simulink model "HSX_double_fin2"  (R2023b)
settings: Solver=VariableStepAuto  StartTime=0.0  StopTime=T_end  RelTol=1e-3
values from neighbouring files (symbols this model uses):
  Kaa = 0    [fin.m]
  Kanti = 0.95    [fin.m]
  Ki = K*Rtot    (= 45.48)    [fin.m]
  Kii = 0.001    [fin.m]
  Kp = K*Ltot    (= 10.10125)    [fin.m]
  Kpp = 0.01    [fin.m]
  Lc = 100e-6    (= 0.0001)    [fin.m]
  LHSX = 0.02    [fin.m]
  Ltot = 10*LHSX+La+Lc/n    (= 0.202025)    [fin.m]
  multi_enable = 1    [fin.m]
  n = 4    [fin.m]
  Ra = 0.0096    [fin.m]
  RHSX = 0.09    [fin.m]
  T_trigger = 15    [fin.m]
  Tdead = Ts/100    (= 1e-06)    [fin.m]
  Ts = 1/fs    (= 0.0001)    [fin.m]
  Tsamp = 1/fsamp    (= 2e-05)    [fin.m]
  VDC = 40    [fin.m]
  Vf = 3.1    [fin.m]
libraries: spsCurrentMeasurementLib x6, spsVoltageMeasurementLib x6, spsSeriesRLCBranchLib x6, spsTriangleGeneratorLib x4, spsMosfetLib x4, spsControlledVoltageSourceLib x2, spsDCMachineLib x2, spsGroundLib x2, spsIdealSwitchLib x2, spsDCVoltageSourceLib x2, spsDiodeLib x1, sps_lib x1
settings Model: Creator=baik3-ad  LastModifiedBy=Hyeongmeen

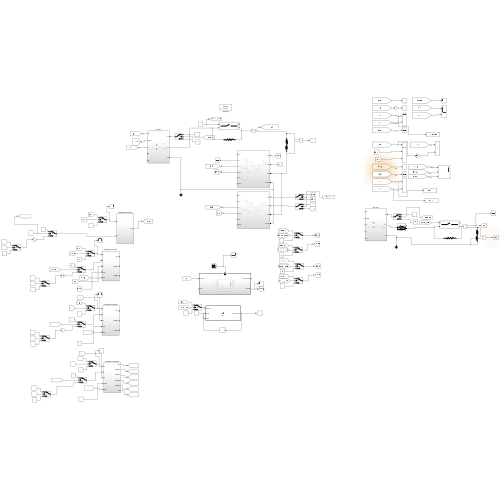
[thumbnail: Simulink's stored preview of the top-level diagram]
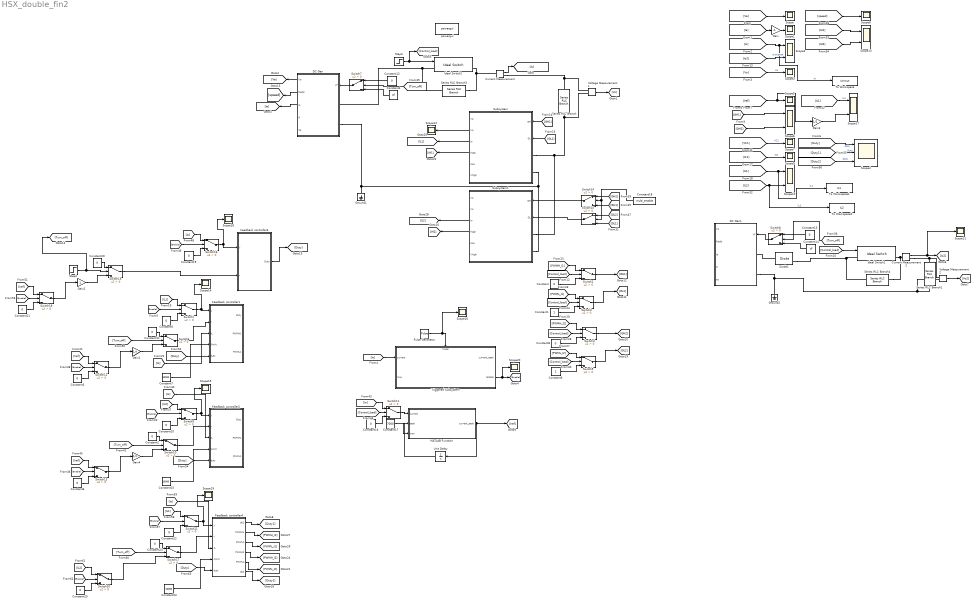
== system HSX_double_fin2 ==
  Constant{,2..3,5..6,8,10..13,16,19..22,24..25} (17 alike) : Constant  Value=0
  Constant1 : Constant
  Constant14 : Constant  Value=Vf
  Constant15 : Constant  Value=10000
  Constant17 : Constant  Value=7000
  Constant18 : Constant  Value=multi_enable
  Constant23 : Constant  Value=10000
  Constant4 : Constant  Value=Vf
  Constant7 : Constant  Value=10000
  Constant9 : Constant
  Current Measurement : spsCurrentMeasurementLib/Current Measurement  PhasorSimulation=off  OutputType=Complex  PSBequivalent=0
  Current Measurement2 : spsCurrentMeasurementLib/Current Measurement  PhasorSimulation=off  OutputType=Complex  PSBequivalent=0
  DC Gen : Subsystem
  DC Gen1 : Subsystem
  Diode1 : spsDiodeLib/Diode  Ron=0.001  Lon=0  Vf=0.8  IC=0  UseSnubber=0  Rs=500  Cs=250e-9  Measurements=on
  Feedback controller1 : Subsystem
  Feedback controller2 : Subsystem
  Feedback controller3 : Subsystem
  Feedback controller4 : Subsystem
  Gain : Gain  Gain=-1
  Gain1 : Gain  Gain=1/n
  Gain2 : Gain
  Gain3 : Gain  Gain=1/2
  Gain4 : Gain  Gain=1/n
  Ground1 : spsGroundLib/Ground  LConnTagsString=a
  Ground2 : spsGroundLib/Ground  LConnTagsString=a
  Ideal Switch1 : spsIdealSwitchLib/Ideal Switch  Ron=1e-6  Lon=0  IC=0  Rs=1e8  Cs=0  Measurements=on
  Ideal Switch2 : spsIdealSwitchLib/Ideal Switch  Ron=1e-6  Lon=0  IC=0  Rs=1e8  Cs=0  Measurements=on
  MATLAB Function : MATLAB Function  TreatAsAtomicUnit=on
  Pulse Generator : DiscretePulseGenerator  PulseType=Time based  Period=Ts  PulseWidth=50
  Scope{,1,3,5,7..9,11..12,14..16,18..20} (15 alike) : Scope
  Scope{2,6,10,13,17} (5 alike) : Scope  NumInputPorts=2
  Scope4 : Scope  NumInputPorts=3
  Series RLC Branch : spsSeriesRLCBranchLib/Series RLC Branch  LConnTagsString=__new0  RConnTagsString=__new0  BranchType=RL  Resistance=RHSX*10  Inductance=LHSX*10  SetiL0=off  InitialCurrent=0  Capacitance=1e-6  Setx0=off  InitialVoltage=0  Measurements=None
  Series RLC Branch1 : spsSeriesRLCBranchLib/Series RLC Branch  LConnTagsString=__new0  RConnTagsString=__new0  BranchType=RL  Resistance=RHSX*10  Inductance=LHSX*10  SetiL0=off  InitialCurrent=0  Capacitance=1e-6  Setx0=off  InitialVoltage=0  Measurements=None
  Series RLC Branch3 : spsSeriesRLCBranchLib/Series RLC Branch  LConnTagsString=__new0  RConnTagsString=__new0  BranchType=R  Resistance=1e8  Inductance=0  SetiL0=off  InitialCurrent=0  Capacitance=1e-6  Setx0=off  InitialVoltage=0  Measurements=None
  Series RLC Branch4 : spsSeriesRLCBranchLib/Series RLC Branch  LConnTagsString=__new0  RConnTagsString=__new0  BranchType=R  Resistance=1e8  Inductance=0  SetiL0=off  InitialCurrent=0  Capacitance=1e-6  Setx0=off  InitialVoltage=0  Measurements=None
  Step2 : Step  Time=T_trigger+1.5  SampleTime=0  VectorParams1D=off  ZeroCross=off
  Step3 : Step  Time=T_trigger  SampleTime=0  VectorParams1D=off  ZeroCross=off
  Subsystem : Subsystem
  Subsystem1 : Subsystem
  Switch{1..21} (21 alike) : Switch  Criteria=u2 > Threshold  SaturateOnIntegerOverflow=off  InputSameDT=off
  To Workspace : ToWorkspace  VariableName=simout  SaveFormat=Timeseries  SampleTime=-1
  To Workspace1 : ToWorkspace  VariableName=IL1  SaveFormat=Timeseries  SampleTime=-1
  To Workspace2 : ToWorkspace  VariableName=IL2  SaveFormat=Timeseries  SampleTime=-1
  Triggered Subsystem : Subsystem  TreatAsAtomicUnit=on
  Unit Delay : UnitDelay  SampleTime=-1  HasFrameUpgradeWarning=on
  Voltage Measurement1 : spsVoltageMeasurementLib/Voltage Measurement  PhasorSimulation=off  OutputType=Complex  PSBequivalent=0
  Voltage Measurement2 : spsVoltageMeasurementLib/Voltage Measurement  PhasorSimulation=off  OutputType=Complex  PSBequivalent=0
  powergui : sps_lib/powergui  Priority=1  SimulationMode=Discrete  SampleTime=Tsamp  frequency=60  Iterations=50  frequencyindice=0  Pbase=100e6  ErrMax=1e-4  UnitsV=kV  UnitsW=MW  buscounter=0  FunctionMessages=off  echomessages=off  EnableUseOfTLC=off  CurrentSourceSwitches=off  DisableSnubberDevices=off  DisableRonSwitches=off  DisableVfSwitches=off  DisplayEquations=off  AutomaticDiscreteSolvers=off  SolverType=Tustin/Backward Euler (TBE)  Interpol=off  ExternalGateDelay=off  methode=off  Ts=100  x0status=blocks  SPID=on  SwTol=0  HookPort=off  NonlinearTolerance=1e-4  nMaxIteration=100  ContinueOnMaxIteration=off  RestoreLinks=warning  ResistiveCurrentMeasurement=off  Frange=[0:2:500]  Ylog=off  Xlog=on  ShowGrid=off  save=off  variable=ZData  structure=0  ZoomFFT=off  StartTime=0.0  cycles=1  DisplayStyle=1  fundamental=60  FreqAxis=off  MaxFrequency=1000  frequencyindicesteady=1  RmsSteady=1  display=off
  wires:
  Step3/1 -> [Control_load], Ideal Switch2/1
  Current Measurement/1 -> [Io]
  Voltage Measurement1/1 -> [Vo]
  [Va] -> Scope/1
  [Io] -> To Workspace/1, Scope2/1  "Io"
  [Vo] -> Scope3/1  "Vo"
  [Ia] -> Gain/1
  Gain/1 -> Scope1/1
  [Iref] -> Gain3/1, Scope5/1
  [VC1] -> Scope7/1  "VC1"
  Switch2/1 -> [GH1]
  Switch3/1 -> [GL1]
  [speed] -> Scope8/1
  [IC1] -> Scope9/1  "IC1"
  [IL1] -> To Workspace1/1, Scope10/1  "IL1"
  [Enable] -> Switch1/2
  Constant5/1 -> Switch1/3
  [IL1] -> Switch1/1
  Switch1/1 -> Feedback controller1/1(y), Scope14/1
  Switch6/1 -> Feedback controller1/2(r)
  [Control_load] -> Switch2/2
  [PWMH_I1] -> Switch2/1
  Constant/1 -> Switch2/3
  [PWML_I1] -> Switch3/1
  Constant1/1 -> Switch3/3
  [Control_load] -> Switch3/2
  Current Measurement2/1 -> Scope11/1, [Io2]
  Voltage Measurement2/1 -> [Vo2]
  [Control_load] -> Ideal Switch1/1
  [Io2] -> Scope2/2  "Io original"
  [Io] -> Feedback controller1/3(IL)
  Constant7/1 -> Feedback controller1/4(Ilimit)
  Switch7/1 -> DC Gen/1(Vf)
  Subsystem/3(Io) -> [IL1]
  Subsystem/2(Vo) -> Scope12/1
  DC Gen/3(Ia) -> [Ia]
  DC Gen/1(Va) -> [Va]
  DC Gen/2(Rad/s) -> [speed]
  Switch4/1 -> [GH2]
  [Control_load] -> Switch5/2
  Constant9/1 -> Switch5/3
  [Control_load] -> Switch4/2
  [PWML_I2] -> Switch5/1
  [PWMH_I2] -> Switch4/1
  Constant8/1 -> Switch4/3
  Switch5/1 -> [GL2]
  [GH1] -> Subsystem/1(GH)
  [IL2] -> To Workspace2/1, Scope10/2  "IL2"
  [IH1] -> Scope13/1
  [IH2] -> Scope13/2
  Subsystem/4(Ihigh) -> [IH1]
  [Turn_off] -> Switch6/2
  Constant11/1 -> Switch6/1
  Constant4/1 -> Switch7/3
  [Turn_off] -> Switch7/2
  Constant12/1 -> Switch7/1
  Constant13/1 -> Switch8/1
  Constant14/1 -> Switch8/3
  [Turn_off] -> Switch8/2
  Switch8/1 -> DC Gen1/1(Vf)
  Switch14/1 -> Subsystem1/1(GH)
  Subsystem1/3(Io) -> [IL2]
  Subsystem1/4(Ihigh) -> [IH2]
  Constant2/1 -> Switch10/1
  [Io] -> Feedback controller2/3(IL)
  Switch9/1 -> Scope15/1, Feedback controller2/1(y)
  [Turn_off] -> Switch10/2
  Constant15/1 -> Feedback controller2/4(Ilimit)
  Switch10/1 -> Feedback controller2/2(r)
  [Enable] -> Switch9/2
  Constant10/1 -> Switch9/3
  [IL2] -> Switch9/1
  Switch12/1 -> Gain1/1
  Gain1/1 -> Switch6/3
  Gain4/1 -> Switch10/3
  Pulse Generator/1 -> Scope16/1, Triggered Subsystem/Trigger
  [IL1] -> Scope17/1  "IL1"
  Gain3/1 -> Scope17/2
  [Control_load] -> Switch11/2
  [Io] -> Switch11/1
  Constant17/1 -> MATLAB Function/3(max)
  Constant16/1 -> Switch11/3
  Switch11/1 -> MATLAB Function/1(current)
  MATLAB Function/1(current_peak) -> Unit Delay/1, [Iref]
  Unit Delay/1 -> MATLAB Function/2(peak)
  [Io] -> Triggered Subsystem/1(current)
  Triggered Subsystem/2(Enable) -> Scope20/1, [Enable]
  [Enable] -> Switch12/2
  [Iref] -> Switch12/1
  Constant3/1 -> Switch12/3
  Constant6/1 -> Switch13/3
  [Iref] -> Switch13/1
  [Enable] -> Switch13/2
  Switch13/1 -> Gain4/1
  Switch15/1 -> Subsystem1/2(GL)
  [GL1] -> Subsystem/2(GL)
  [GH1] -> Scope6/1
  [GH2] -> Scope6/2
  [GH2] -> Switch14/1
  [GL2] -> Switch15/1
  [GH1] -> Switch14/3
  [GL1] -> Switch15/3
  Constant18/1 -> Switch15/2, Switch14/2
  [Enable] -> Switch16/2
  [Io] -> Switch16/1
  Switch16/1 -> Feedback controller3/1(y), Scope18/1
  Constant19/1 -> Switch16/3
  Switch19/1 -> Feedback controller3/2(r)
  [Enable] -> Switch18/2
  Constant21/1 -> Switch18/3
  Gain2/1 -> Switch19/3
  Switch18/1 -> Gain2/1
  [Iref] -> Switch18/1
  Step2/1 -> [Turn_off], Switch19/2
  Constant20/1 -> Switch19/1
  Feedback controller3/1(Duty) -> [Duty]
  [Duty] -> Feedback controller1/5(duty)
  [Duty] -> Feedback controller2/5(duty)
  [Duty] -> Scope4/1  "Duty"
  [Duty1] -> Scope4/2  "Duty"
  [Duty2] -> Scope4/3  "Duty"
  Constant24/1 -> Switch17/1
  [Turn_off] -> Switch17/2
  Constant25/1 -> Switch20/3
  Switch20/1 -> Switch17/3
  [Duty] -> Feedback controller4/5(duty)
  [Enable] -> Switch20/2
  [IL2] -> Switch20/1
  Constant23/1 -> Feedback controller4/4(Ilimit)
  Constant22/1 -> Switch21/3
  [IL1] -> Switch21/1
  Switch21/1 -> Scope19/1, Feedback controller4/1(y)
  Switch17/1 -> Feedback controller4/2(r)
  [Enable] -> Switch21/2
  [Io] -> Feedback controller4/3(IL)
  Feedback controller4/4(PWMH2) -> [PWMH_I2]
  Feedback controller4/5(PWML2) -> [PWML_I2]
  Feedback controller4/3(PWML1) -> [PWML_I1]
  Feedback controller4/2(PWMH1) -> [PWMH_I1]
  Feedback controller4/1(do1) -> [Duty1]
  Feedback controller4/6(do2) -> [Duty2]
  connections:
  DC Gen/LConn2 -- Subsystem1/LConn2 -- Subsystem/LConn2 -- Ground1/LConn1
  Current Measurement/RConn1 -- Voltage Measurement1/LConn1 -- Series RLC Branch/LConn1
  Current Measurement/LConn1 -- Ideal Switch2/RConn1 -- Series RLC Branch3/LConn1
  Ideal Switch1/LConn1 -- Diode1/RConn1 -- Series RLC Branch4/RConn1
  Ideal Switch1/RConn1 -- Current Measurement2/LConn1 -- Series RLC Branch4/LConn1
  Series RLC Branch1/LConn1 -- Voltage Measurement2/LConn1 -- Current Measurement2/RConn1
  Diode1/LConn1 -- DC Gen1/LConn1
  DC Gen1/LConn2 -- Series RLC Branch1/RConn1 -- Voltage Measurement2/LConn2 -- Ground2/LConn1
  Ideal Switch2/LConn1 -- DC Gen/LConn1 -- Series RLC Branch3/RConn1
  Voltage Measurement1/LConn2 -- Subsystem1/LConn1 -- Subsystem/LConn1 -- Series RLC Branch/RConn1

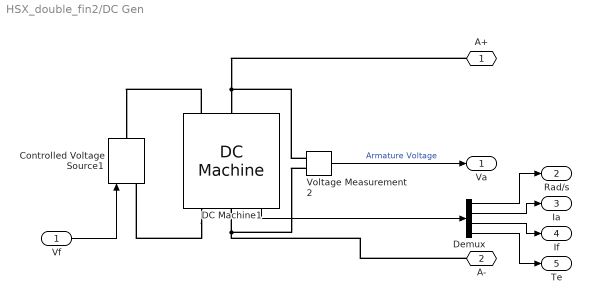
== system HSX_double_fin2/DC Gen ==
  Vf : Inport
  Controlled Voltage Source1 : spsControlledVoltageSourceLib/Controlled Voltage Source  Initialize=on  Source_Type=DC  Amplitude=0  Phase=0  Frequency=0  Measurements=Voltage
  DC Machine1 : spsDCMachineLib/DC Machine  PresetModel=No  MechanicalLoad=Torque TL  FieldType=Wound  ShowDetailedParameters=on  MeasurementBus=off  RLa="[Ra  0.002]"  RLf=[0.0054 0.0125]  Laf=Laf  MachineConstant=Torque constant (N.m/A)  Ke=1.8  Kt=1.8  J=137  Bm=0  Tf=0  w0=w_initial  Ifinit=0  TsPowergui=0  TsBlock=-1
  Demux : Demux
  Voltage Measurement2 : spsVoltageMeasurementLib/Voltage Measurement  PhasorSimulation=off  OutputType=Complex  PSBequivalent=0
  A+ : PMIOPort  Side=Left
  A- : PMIOPort  Port=2  Side=Left
  Va : Outport
  Rad/s : Outport  Port=2
  Ia : Outport  Port=3
  If : Outport  Port=4
  Te : Outport  Port=5
  wires:
  DC Machine1/1 -> Demux/1
  Vf/1 -> Controlled Voltage Source1/1
  Voltage Measurement2/1 -> Va/1  "Armature Voltage"
  Demux/1 -> Rad/s/1
  Demux/4 -> Te/1
  Demux/3 -> If/1
  Demux/2 -> Ia/1
  connections:
  Voltage Measurement2/LConn1 -- A+/RConn1 -- DC Machine1/LConn1
  A-/RConn1 -- Voltage Measurement2/LConn2 -- DC Machine1/RConn1
  DC Machine1/LConn2 -- Controlled Voltage Source1/RConn1
  DC Machine1/RConn2 -- Controlled Voltage Source1/LConn1

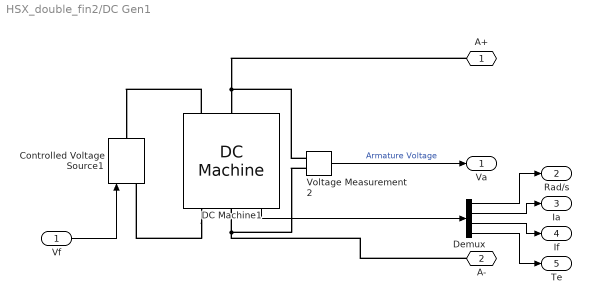
== system HSX_double_fin2/DC Gen1 ==
  Vf : Inport
  Controlled Voltage Source1 : spsControlledVoltageSourceLib/Controlled Voltage Source  Initialize=on  Source_Type=DC  Amplitude=0  Phase=0  Frequency=0  Measurements=Voltage
  DC Machine1 : spsDCMachineLib/DC Machine  PresetModel=No  MechanicalLoad=Torque TL  FieldType=Wound  ShowDetailedParameters=on  MeasurementBus=off  RLa="[Ra  0.002]"  RLf=[0.0054 0.0125]  Laf=Laf  MachineConstant=Torque constant (N.m/A)  Ke=1.8  Kt=1.8  J=137  Bm=0  Tf=0  w0=w_initial  Ifinit=0  TsPowergui=0  TsBlock=-1
  Demux : Demux
  Voltage Measurement2 : spsVoltageMeasurementLib/Voltage Measurement  PhasorSimulation=off  OutputType=Complex  PSBequivalent=0
  A+ : PMIOPort  Side=Left
  A- : PMIOPort  Port=2  Side=Left
  Va : Outport
  Rad/s : Outport  Port=2
  Ia : Outport  Port=3
  If : Outport  Port=4
  Te : Outport  Port=5
  wires:
  DC Machine1/1 -> Demux/1
  Vf/1 -> Controlled Voltage Source1/1
  Voltage Measurement2/1 -> Va/1  "Armature Voltage"
  Demux/1 -> Rad/s/1
  Demux/4 -> Te/1
  Demux/3 -> If/1
  Demux/2 -> Ia/1
  connections:
  Voltage Measurement2/LConn1 -- A+/RConn1 -- DC Machine1/LConn1
  A-/RConn1 -- Voltage Measurement2/LConn2 -- DC Machine1/RConn1
  DC Machine1/LConn2 -- Controlled Voltage Source1/RConn1
  DC Machine1/RConn2 -- Controlled Voltage Source1/LConn1

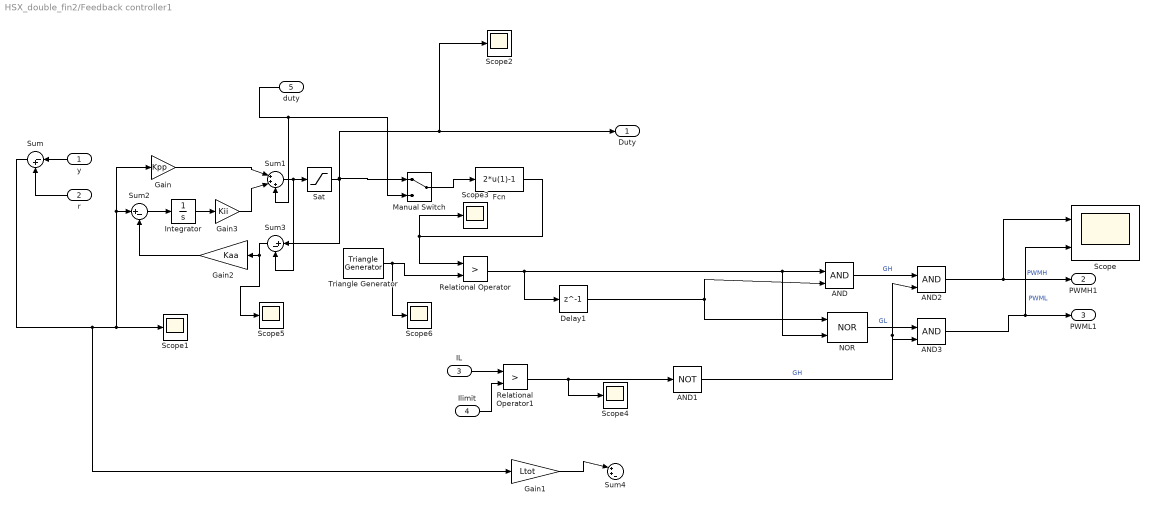
== system HSX_double_fin2/Feedback controller1 ==
  y : Inport
  r : Inport  Port=2
  IL : Inport  Port=3
  Ilimit : Inport  Port=4
  duty : Inport  Port=5
  AND : Logic  IconShape=distinctive  AllPortsSameDT=off  OutDataTypeStr=boolean
  AND1 : Logic  Operator=NOT  IconShape=distinctive  AllPortsSameDT=off  OutDataTypeStr=boolean
  AND2 : Logic  IconShape=distinctive  AllPortsSameDT=off  OutDataTypeStr=boolean
  AND3 : Logic  IconShape=distinctive  AllPortsSameDT=off  OutDataTypeStr=boolean
  Delay1 : Delay  DelayLength=1  InitialCondition=0  SampleTime=Tdead
  Fcn : Fcn  Expr=2*u(1)-1
  Gain : Gain  Gain=Kpp
  Gain1 : Gain  Gain=Ltot
  Gain2 : Gain  Gain=Kaa
  Gain3 : Gain  Gain=Kii
  Integrator : Integrator
  Manual Switch : ManualSwitch
  NOR : Logic  Operator=NOR  IconShape=distinctive  AllPortsSameDT=off
  Relational Operator : RelationalOperator  Operator=>  OutDataTypeStr=boolean  RndMeth=Simplest  InputSameDT=off
  Relational Operator1 : RelationalOperator  Operator=>  OutDataTypeStr=boolean  RndMeth=Simplest  InputSameDT=off
  Sat : Saturate  UpperLimit=1  LowerLimit=0
  Scope : Scope  NumInputPorts=2
  Scope{1..6} (6 alike) : Scope
  Sum : Sum  Inputs=|-+  InputSameDT=on  SaturateOnIntegerOverflow=on  OutDataTypeStr=Inherit: Same as first input
  Sum1 : Sum  Inputs=|+++
  Sum2 : Sum  Inputs=|+-
  Sum3 : Sum  Inputs=|+-
  Sum4 : Sum  Inputs=|++-
  Triangle Generator : spsTriangleGeneratorLib/Triangle Generator  Freq=1/Ts  Phase=0  Ts=Tsamp
  Duty : Outport  VectorParamsAs1DForOutWhenUnconnected=off
  PWMH1 : Outport  Port=2  VectorParamsAs1DForOutWhenUnconnected=off
  PWML1 : Outport  Port=3  VectorParamsAs1DForOutWhenUnconnected=off
  wires:
  Sum/1 -> Gain1/1, Scope1/1, Gain/1, Sum2/1
  y/1 -> Sum/1
  r/1 -> Sum/2
  Sat/1 -> Sum3/1, Manual Switch/1, Scope2/1, Duty/1
  Sum1/1 -> Sum3/2, Sat/1
  Gain/1 -> Sum1/1
  Sum2/1 -> Integrator/1
  Sum3/1 -> Scope5/1, Gain2/1
  Gain2/1 -> Sum2/2
  Triangle Generator/1 -> Scope6/1, Relational Operator/2
  Relational Operator/1 -> Delay1/1, NOR/2, AND/1
  Delay1/1 -> NOR/1, AND/2
  Fcn/1 -> Scope3/1, Relational Operator/1
  Integrator/1 -> Gain3/1
  Gain3/1 -> Sum1/2
  IL/1 -> Relational Operator1/1
  Ilimit/1 -> Relational Operator1/2
  AND/1 -> AND2/1  "GH"
  AND2/1 -> Scope/1, PWMH1/1  "PWMH"
  AND3/1 -> PWML1/1, Scope/2  "PWML"
  NOR/1 -> AND3/1  "GL"
  Relational Operator1/1 -> Scope4/1, AND1/1
  AND1/1 -> AND3/2, AND2/2  "GH"
  Manual Switch/1 -> Fcn/1
  Gain1/1 -> Sum4/1
  duty/1 -> Sum1/3, Manual Switch/2

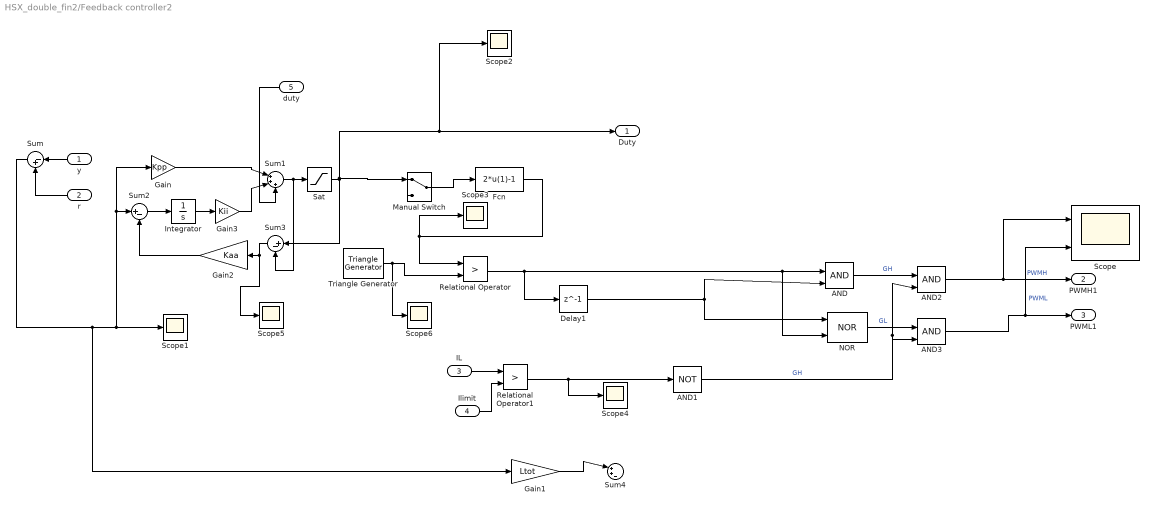
== system HSX_double_fin2/Feedback controller2 ==
  y : Inport
  r : Inport  Port=2
  IL : Inport  Port=3
  Ilimit : Inport  Port=4
  duty : Inport  Port=5
  AND : Logic  IconShape=distinctive  AllPortsSameDT=off  OutDataTypeStr=boolean
  AND1 : Logic  Operator=NOT  IconShape=distinctive  AllPortsSameDT=off  OutDataTypeStr=boolean
  AND2 : Logic  IconShape=distinctive  AllPortsSameDT=off  OutDataTypeStr=boolean
  AND3 : Logic  IconShape=distinctive  AllPortsSameDT=off  OutDataTypeStr=boolean
  Delay1 : Delay  DelayLength=1  InitialCondition=0  SampleTime=Tdead
  Fcn : Fcn  Expr=2*u(1)-1
  Gain : Gain  Gain=Kpp
  Gain1 : Gain  Gain=Ltot
  Gain2 : Gain  Gain=Kaa
  Gain3 : Gain  Gain=Kii
  Integrator : Integrator
  Manual Switch : ManualSwitch
  NOR : Logic  Operator=NOR  IconShape=distinctive  AllPortsSameDT=off
  Relational Operator : RelationalOperator  Operator=>  OutDataTypeStr=boolean  RndMeth=Simplest  InputSameDT=off
  Relational Operator1 : RelationalOperator  Operator=>  OutDataTypeStr=boolean  RndMeth=Simplest  InputSameDT=off
  Sat : Saturate  UpperLimit=1  LowerLimit=0
  Scope : Scope  NumInputPorts=2
  Scope{1..6} (6 alike) : Scope
  Sum : Sum  Inputs=|-+  InputSameDT=on  SaturateOnIntegerOverflow=on  OutDataTypeStr=Inherit: Same as first input
  Sum1 : Sum  Inputs=|+++
  Sum2 : Sum  Inputs=|+-
  Sum3 : Sum  Inputs=|+-
  Sum4 : Sum  Inputs=|++-
  Triangle Generator : spsTriangleGeneratorLib/Triangle Generator  Freq=1/Ts  Phase=180  Ts=Tsamp
  Duty : Outport  VectorParamsAs1DForOutWhenUnconnected=off
  PWMH1 : Outport  Port=2  VectorParamsAs1DForOutWhenUnconnected=off
  PWML1 : Outport  Port=3  VectorParamsAs1DForOutWhenUnconnected=off
  wires:
  Sum/1 -> Gain1/1, Scope1/1, Gain/1, Sum2/1
  y/1 -> Sum/1
  r/1 -> Sum/2
  Sat/1 -> Sum3/1, Manual Switch/1, Scope2/1, Duty/1
  Sum1/1 -> Sum3/2, Sat/1
  Gain/1 -> Sum1/1
  Sum2/1 -> Integrator/1
  Sum3/1 -> Scope5/1, Gain2/1
  Gain2/1 -> Sum2/2
  Triangle Generator/1 -> Scope6/1, Relational Operator/2
  Relational Operator/1 -> Delay1/1, NOR/2, AND/1
  Delay1/1 -> NOR/1, AND/2
  Fcn/1 -> Scope3/1, Relational Operator/1
  Integrator/1 -> Gain3/1
  Gain3/1 -> Sum1/2
  IL/1 -> Relational Operator1/1
  Ilimit/1 -> Relational Operator1/2
  AND/1 -> AND2/1  "GH"
  AND2/1 -> Scope/1, PWMH1/1  "PWMH"
  AND3/1 -> PWML1/1, Scope/2  "PWML"
  NOR/1 -> AND3/1  "GL"
  Relational Operator1/1 -> Scope4/1, AND1/1
  AND1/1 -> AND3/2, AND2/2  "GH"
  Manual Switch/1 -> Fcn/1
  Gain1/1 -> Sum4/1
  duty/1 -> Sum1/3

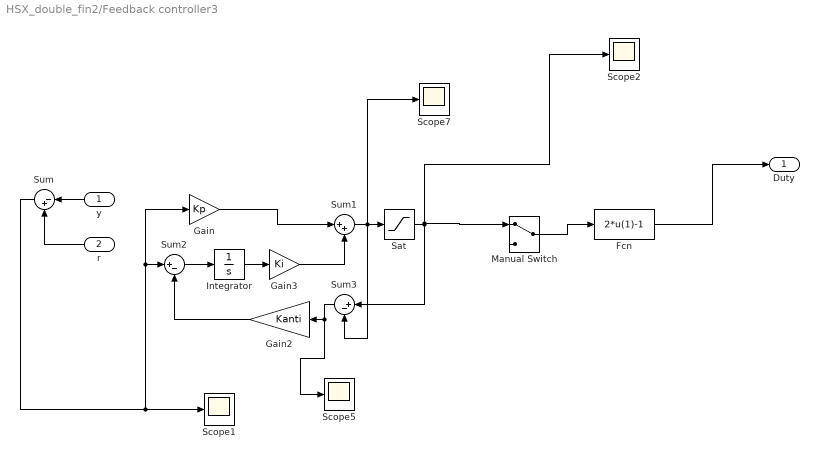
== system HSX_double_fin2/Feedback controller3 ==
  y : Inport
  r : Inport  Port=2
  Fcn : Fcn  Expr=2*u(1)-1
  Gain : Gain  Gain=Kp
  Gain2 : Gain  Gain=Kanti
  Gain3 : Gain  Gain=Ki
  Integrator : Integrator
  Manual Switch : ManualSwitch
  Sat : Saturate  UpperLimit=1  LowerLimit=0
  Scope{1..2,5,7} (4 alike) : Scope
  Sum : Sum  Inputs=|-+  InputSameDT=on  SaturateOnIntegerOverflow=on  OutDataTypeStr=Inherit: Same as first input
  Sum1 : Sum  Inputs=|++
  Sum2 : Sum  Inputs=|+-
  Sum3 : Sum  Inputs=|+-
  Duty : Outport  VectorParamsAs1DForOutWhenUnconnected=off
  wires:
  Sum/1 -> Scope1/1, Gain/1, Sum2/1
  y/1 -> Sum/1
  r/1 -> Sum/2
  Sat/1 -> Sum3/1, Manual Switch/1, Scope2/1
  Gain/1 -> Sum1/1
  Sum2/1 -> Integrator/1
  Sum3/1 -> Scope5/1, Gain2/1
  Gain2/1 -> Sum2/2
  Integrator/1 -> Gain3/1
  Gain3/1 -> Sum1/2
  Manual Switch/1 -> Fcn/1
  Sum1/1 -> Scope7/1, Sat/1, Sum3/2
  Fcn/1 -> Duty/1

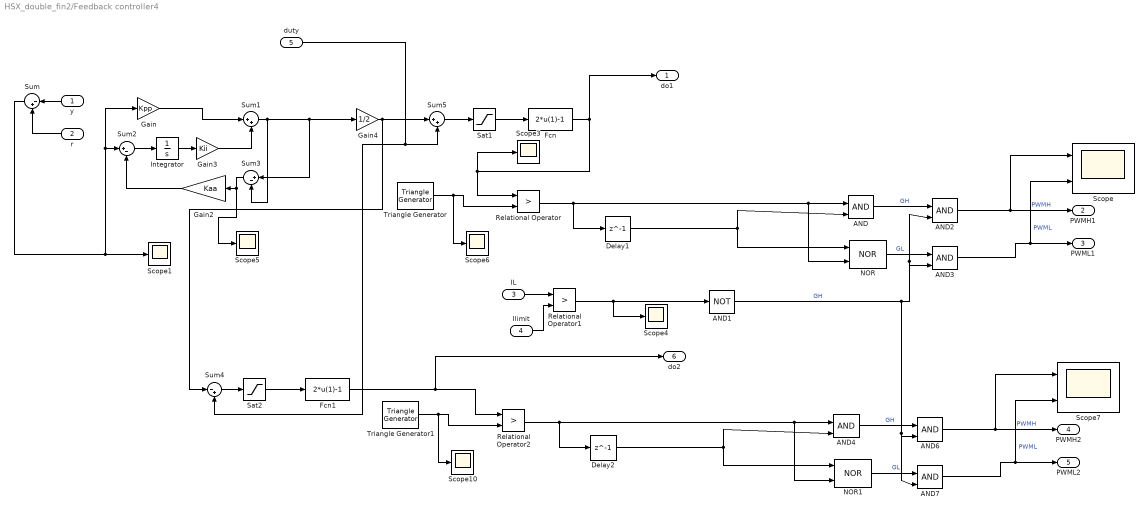
== system HSX_double_fin2/Feedback controller4 ==
  y : Inport
  r : Inport  Port=2
  IL : Inport  Port=3
  Ilimit : Inport  Port=4
  duty : Inport  Port=5
  AND{,2..4,6..7} (6 alike) : Logic  IconShape=distinctive  AllPortsSameDT=off  OutDataTypeStr=boolean
  AND1 : Logic  Operator=NOT  IconShape=distinctive  AllPortsSameDT=off  OutDataTypeStr=boolean
  Delay1 : Delay  DelayLength=1  InitialCondition=0  SampleTime=Tdead
  Delay2 : Delay  DelayLength=1  InitialCondition=0  SampleTime=Tdead
  Fcn : Fcn  Expr=2*u(1)-1
  Fcn1 : Fcn  Expr=2*u(1)-1
  Gain : Gain  Gain=Kpp
  Gain2 : Gain  Gain=Kaa
  Gain3 : Gain  Gain=Kii
  Gain4 : Gain  Gain=1/2
  Integrator : Integrator
  NOR : Logic  Operator=NOR  IconShape=distinctive  AllPortsSameDT=off
  NOR1 : Logic  Operator=NOR  IconShape=distinctive  AllPortsSameDT=off
  Relational Operator : RelationalOperator  Operator=>  OutDataTypeStr=boolean  RndMeth=Simplest  InputSameDT=off
  Relational Operator1 : RelationalOperator  Operator=>  OutDataTypeStr=boolean  RndMeth=Simplest  InputSameDT=off
  Relational Operator2 : RelationalOperator  Operator=>  OutDataTypeStr=boolean  RndMeth=Simplest  InputSameDT=off
  Sat1 : Saturate  UpperLimit=1  LowerLimit=0
  Sat2 : Saturate  UpperLimit=1  LowerLimit=0
  Scope : Scope  NumInputPorts=2
  Scope{1,3..6,10} (6 alike) : Scope
  Scope7 : Scope  NumInputPorts=2
  Sum : Sum  Inputs=|-+  InputSameDT=on  SaturateOnIntegerOverflow=on  OutDataTypeStr=Inherit: Same as first input
  Sum1 : Sum  Inputs=|++
  Sum2 : Sum  Inputs=|+-
  Sum3 : Sum  Inputs=|+-
  Sum4 : Sum  Inputs=|-+
  Sum5 : Sum  Inputs=|++
  Triangle Generator : spsTriangleGeneratorLib/Triangle Generator  Freq=1/Ts  Phase=0  Ts=Tsamp
  Triangle Generator1 : spsTriangleGeneratorLib/Triangle Generator  Freq=1/Ts  Phase=180  Ts=Tsamp
  do1 : Outport  VectorParamsAs1DForOutWhenUnconnected=off
  PWMH1 : Outport  Port=2  VectorParamsAs1DForOutWhenUnconnected=off
  PWML1 : Outport  Port=3  VectorParamsAs1DForOutWhenUnconnected=off
  PWMH2 : Outport  Port=4  VectorParamsAs1DForOutWhenUnconnected=off
  PWML2 : Outport  Port=5  VectorParamsAs1DForOutWhenUnconnected=off
  do2 : Outport  Port=6  VectorParamsAs1DForOutWhenUnconnected=off
  wires:
  Sum/1 -> Scope1/1, Gain/1, Sum2/1
  y/1 -> Sum/1
  r/1 -> Sum/2
  Sum1/1 -> Gain4/1, Sum3/1, Sum3/2
  Gain/1 -> Sum1/1
  Sum2/1 -> Integrator/1
  Sum3/1 -> Scope5/1, Gain2/1
  Gain2/1 -> Sum2/2
  Triangle Generator/1 -> Scope6/1, Relational Operator/2
  Relational Operator/1 -> Delay1/1, NOR/2, AND/1
  Delay1/1 -> NOR/1, AND/2
  Fcn/1 -> Scope3/1, Relational Operator/1, do1/1
  Integrator/1 -> Gain3/1
  Gain3/1 -> Sum1/2
  IL/1 -> Relational Operator1/1
  Ilimit/1 -> Relational Operator1/2
  AND/1 -> AND2/1  "GH"
  AND2/1 -> Scope/1, PWMH1/1  "PWMH"
  AND3/1 -> PWML1/1, Scope/2  "PWML"
  NOR/1 -> AND3/1  "GL"
  Relational Operator1/1 -> Scope4/1, AND1/1
  AND1/1 -> AND7/2, AND6/2, AND3/2, AND2/2  "GH"
  Sat1/1 -> Fcn/1
  Sum5/1 -> Sat1/1
  duty/1 -> Sum4/2, Sum5/2
  Gain4/1 -> Sum4/1, Sum5/1
  AND6/1 -> Scope7/1, PWMH2/1  "PWMH"
  AND4/1 -> AND6/1  "GH"
  NOR1/1 -> AND7/1  "GL"
  AND7/1 -> PWML2/1, Scope7/2  "PWML"
  Delay2/1 -> NOR1/1, AND4/2
  Relational Operator2/1 -> Delay2/1, NOR1/2, AND4/1
  Triangle Generator1/1 -> Scope10/1, Relational Operator2/2
  Sat2/1 -> Fcn1/1
  Sum4/1 -> Sat2/1
  Fcn1/1 -> do2/1, Relational Operator2/1

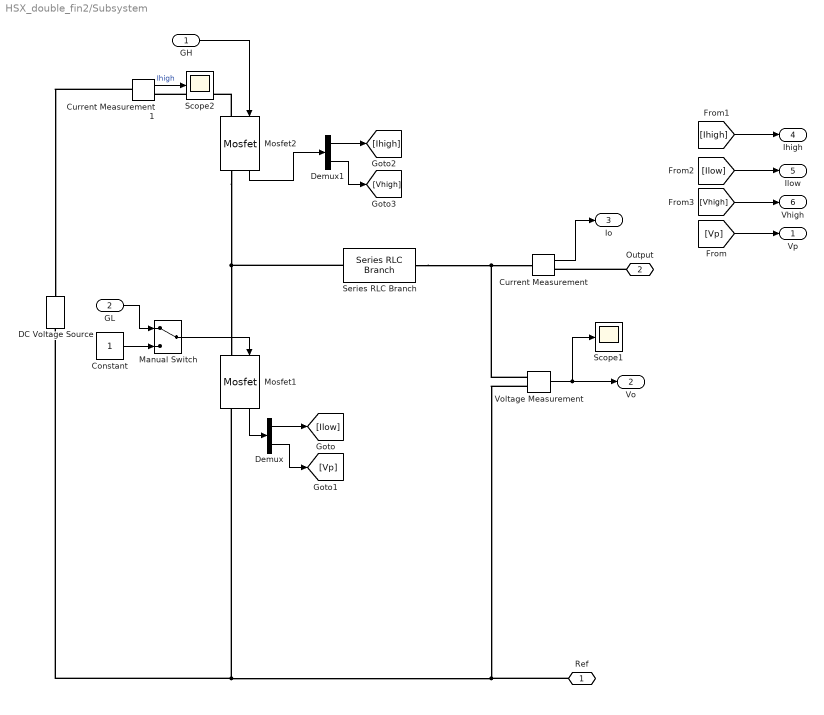
== system HSX_double_fin2/Subsystem ==
  GH : Inport
  GL : Inport  Port=2
  Constant : Constant
  Current Measurement : spsCurrentMeasurementLib/Current Measurement  PhasorSimulation=off  OutputType=Complex  PSBequivalent=0
  Current Measurement1 : spsCurrentMeasurementLib/Current Measurement  PhasorSimulation=off  OutputType=Complex  PSBequivalent=0
  DC Voltage Source : spsDCVoltageSourceLib/DC Voltage Source  Amplitude=VDC  Measurements=None
  Demux : Demux  Outputs=2
  Demux1 : Demux  Outputs=2
  Manual Switch : ManualSwitch
  Mosfet1 : spsMosfetLib/Mosfet  Ron=0.000001  Lon=0  Rd=0.001  Vfd=0.01  IC=0  Rs=1e5  Cs=inf  Measurements=on
  Mosfet2 : spsMosfetLib/Mosfet  Ron=0.000001  Lon=0  Rd=0.001  Vfd=0.01  IC=0  Rs=1e5  Cs=inf  Measurements=on
  Scope1 : Scope
  Scope2 : Scope
  Series RLC Branch : spsSeriesRLCBranchLib/Series RLC Branch  LConnTagsString=__new0  RConnTagsString=__new0  BranchType=L  Resistance=RHSX*10  Inductance=Lc  SetiL0=off  InitialCurrent=0  Capacitance=1e-6  Setx0=off  InitialVoltage=0  Measurements=None
  Voltage Measurement : spsVoltageMeasurementLib/Voltage Measurement  PhasorSimulation=off  OutputType=Complex  PSBequivalent=0
  Ref : PMIOPort  Side=Left
  Output : PMIOPort  Port=2  Side=Left
  Vp : Outport
  Vo : Outport  Port=2
  Io : Outport  Port=3
  Ihigh : Outport  Port=4
  Ilow : Outport  Port=5
  Vhigh : Outport  Port=6
  wires:
  Voltage Measurement/1 -> Vo/1, Scope1/1
  Manual Switch/1 -> Mosfet1/1
  Current Measurement/1 -> Io/1
  Mosfet1/1 -> Demux/1
  Demux/1 -> [Ilow]
  Demux/2 -> [Vp]
  [Vp] -> Vp/1
  GH/1 -> Mosfet2/1
  Demux1/2 -> [Vhigh]
  Mosfet2/1 -> Demux1/1
  Demux1/1 -> [Ihigh]
  [Ihigh] -> Ihigh/1
  [Ilow] -> Ilow/1
  [Vhigh] -> Vhigh/1
  Current Measurement1/1 -> Scope2/1  "Ihigh"
  Constant/1 -> Manual Switch/2
  GL/1 -> Manual Switch/1
  connections:
  Mosfet2/RConn1 -- Series RLC Branch/LConn1 -- Mosfet1/LConn1
  Voltage Measurement/LConn2 -- DC Voltage Source/LConn1 -- Mosfet1/RConn1 -- Ref/RConn1
  Output/RConn1 -- Current Measurement/RConn1
  Current Measurement1/LConn1 -- DC Voltage Source/RConn1
  Mosfet2/LConn1 -- Current Measurement1/RConn1
  Voltage Measurement/LConn1 -- Current Measurement/LConn1 -- Series RLC Branch/RConn1

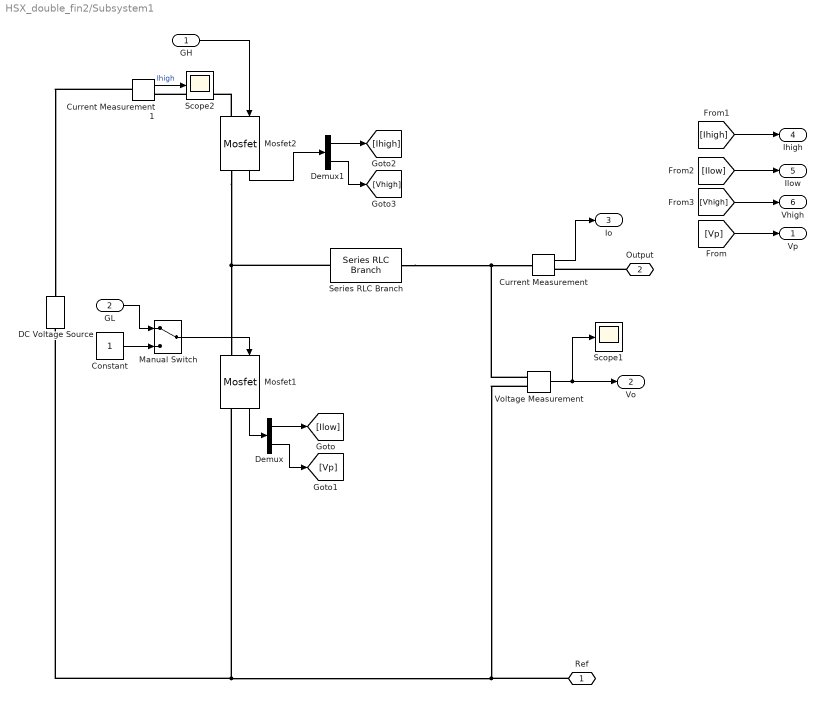
== system HSX_double_fin2/Subsystem1 ==
  GH : Inport
  GL : Inport  Port=2
  Constant : Constant
  Current Measurement : spsCurrentMeasurementLib/Current Measurement  PhasorSimulation=off  OutputType=Complex  PSBequivalent=0
  Current Measurement1 : spsCurrentMeasurementLib/Current Measurement  PhasorSimulation=off  OutputType=Complex  PSBequivalent=0
  DC Voltage Source : spsDCVoltageSourceLib/DC Voltage Source  Amplitude=VDC  Measurements=None
  Demux : Demux  Outputs=2
  Demux1 : Demux  Outputs=2
  Manual Switch : ManualSwitch
  Mosfet1 : spsMosfetLib/Mosfet  Ron=0.000001  Lon=0  Rd=0.001  Vfd=0.01  IC=0  Rs=1e5  Cs=inf  Measurements=on
  Mosfet2 : spsMosfetLib/Mosfet  Ron=0.000001  Lon=0  Rd=0.001  Vfd=0.01  IC=0  Rs=1e5  Cs=inf  Measurements=on
  Scope1 : Scope
  Scope2 : Scope
  Series RLC Branch : spsSeriesRLCBranchLib/Series RLC Branch  LConnTagsString=__new0  RConnTagsString=__new0  BranchType=L  Resistance=RHSX*10  Inductance=Lc  SetiL0=off  InitialCurrent=0  Capacitance=1e-6  Setx0=off  InitialVoltage=0  Measurements=None
  Voltage Measurement : spsVoltageMeasurementLib/Voltage Measurement  PhasorSimulation=off  OutputType=Complex  PSBequivalent=0
  Ref : PMIOPort  Side=Left
  Output : PMIOPort  Port=2  Side=Left
  Vp : Outport
  Vo : Outport  Port=2
  Io : Outport  Port=3
  Ihigh : Outport  Port=4
  Ilow : Outport  Port=5
  Vhigh : Outport  Port=6
  wires:
  Voltage Measurement/1 -> Vo/1, Scope1/1
  Manual Switch/1 -> Mosfet1/1
  Current Measurement/1 -> Io/1
  Mosfet1/1 -> Demux/1
  Demux/1 -> [Ilow]
  Demux/2 -> [Vp]
  [Vp] -> Vp/1
  GH/1 -> Mosfet2/1
  Demux1/2 -> [Vhigh]
  Mosfet2/1 -> Demux1/1
  Demux1/1 -> [Ihigh]
  [Ihigh] -> Ihigh/1
  [Ilow] -> Ilow/1
  [Vhigh] -> Vhigh/1
  Current Measurement1/1 -> Scope2/1  "Ihigh"
  Constant/1 -> Manual Switch/2
  GL/1 -> Manual Switch/1
  connections:
  Mosfet2/RConn1 -- Series RLC Branch/LConn1 -- Mosfet1/LConn1
  Voltage Measurement/LConn2 -- DC Voltage Source/LConn1 -- Mosfet1/RConn1 -- Ref/RConn1
  Output/RConn1 -- Current Measurement/RConn1
  Current Measurement1/LConn1 -- DC Voltage Source/RConn1
  Mosfet2/LConn1 -- Current Measurement1/RConn1
  Voltage Measurement/LConn1 -- Series RLC Branch/RConn1 -- Current Measurement/LConn1

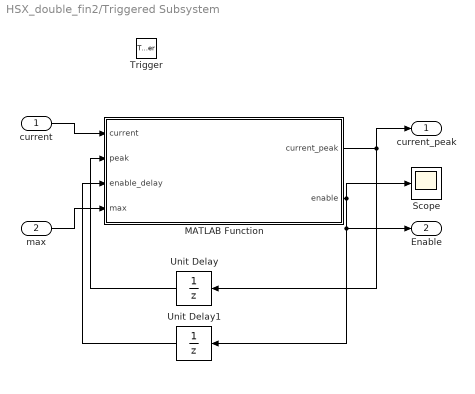
== system HSX_double_fin2/Triggered Subsystem ==
  current : Inport
  max : Inport  Port=2
  Trigger : TriggerPort  TriggerType=either  VariantControl=(inherit)
  MATLAB Function : MATLAB Function  TreatAsAtomicUnit=on
  Scope : Scope
  Unit Delay : UnitDelay  SampleTime=-1  HasFrameUpgradeWarning=on
  Unit Delay1 : UnitDelay  SampleTime=-1  HasFrameUpgradeWarning=on
  current_peak : Outport
  Enable : Outport  Port=2
  wires:
  current/1 -> MATLAB Function/1(current)
  Unit Delay/1 -> MATLAB Function/2(peak)
  max/1 -> MATLAB Function/4(max)
  MATLAB Function/1(current_peak) -> current_peak/1, Unit Delay/1
  MATLAB Function/2(enable) -> Enable/1, Unit Delay1/1, Scope/1
  Unit Delay1/1 -> MATLAB Function/3(enable_delay)

== matlab function HSX_double_fin2/Triggered Subsystem/MATLAB Function ==
  data: current input; current_peak output; peak input; enable_delay input; max input; enable output
function [current_peak, enable] = fcn(current,peak,enable_delay, max)
    if current>peak
        current_peak = current;
    else
        current_peak = peak;
    end

    if (max ~= 0)&&(peak>=max)
        current_peak = max;
     
    end
    
    if enable_delay == 1
        enable = 1;
    else

        if current<peak
            enable = 1;
        else
            enable = 0;
        end
    end

== matlab function HSX_double_fin2/MATLAB Function ==
  data: current input; current_peak output; peak input; max input
function current_peak  = fcn(current,peak,max)
    if current>peak
        current_peak = current;
    else
        current_peak = peak;
    end

    if (max ~= 0)&&(peak>=max)
        current_peak = max;
     
    end
